simulink library "NMEA"  (R2024a)
settings: Solver=VariableStepAuto  StartTime=0.0  StopTime=10.0  RelTol=1e-3
libraries: $bdroot x44, simulink x21, simulink_extras x17, etargetslib x14
(part 1 of 4)
settings Model: Creator=Scythe  LastModifiedBy=Scythe
settings SolverCC: AlgebraicLoopSolver=TrustRegion
settings DataIOCC: ReturnWorkspaceOutputs=off
settings OptimizationCC: ReuseModelBlockBuffer=off
settings DebuggingCC: UnconnectedInputMsg=warning  UnconnectedOutputMsg=warning  UnconnectedLineMsg=warning  ArithmeticOperatorsInVariantConditions=warning
settings ModelReferenceCC: EnableRefExpFcnMdlSchedulingChecks=on
settings SFSimCC: CustomCodeUndefinedFunction=UseInterfaceOnly
settings RTWCC: GPUComputeCapability=3.5  DLArmComputeVersion=19.05

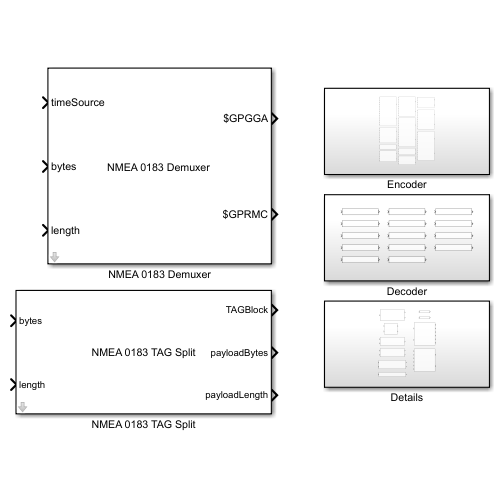
[thumbnail: Simulink's stored preview of the top-level diagram]
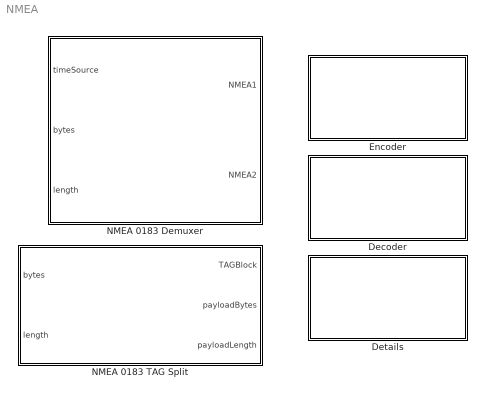
== system NMEA ==
  Decoder : Subsystem
  Details : Subsystem
  Encoder : Subsystem
  NMEA 0183 Demuxer : Subsystem  mask{numMessages=2, idStrings='GPGGA,GPRMC', bufferSize=128, ignoreChecksum=off}
      mask prompts: idStrings "ID strings (separated by comma, e.g: 'GPGGA,GPRMC'):"; bufferSize "Buffer Size (at least 16):"; ignoreChecksum "Ignore Checksum"
      mask help:
      | Receive a binary stream of NMEA 0183 messages and sort them based on the ID. For each ID a separate output port is created. The ID is a string that follows after the start delimiter character.<br><br>
      |
      | <b>timeSource</b><br>
      | The time source to be used to set timestamp values for received messages.<br><br>
      |
      | <b>bytes</b><br>
      | An array of bytes containing binary stream data.<br><br>
      |
      | <b>length</b><br>
      | The length of the actual message in the binary stream data vector.<br><br>
      |
      | <b>OUTPUT PORTS</b><br>
      | An output port is created for each ID string that is specified in the block mask. Each output contains an 8-byte timestamp (double) followed by a buffer containing the actual NMEA message. Thus the output dimension is (8+bufferSize)-by-1. The corresponding output buffer is updated if the checksum is valid or is ignored.
      mask init:
      | % ~~~~~~~~~~~~~~~~~~~~~~~~~~~~~~~~~~~~~~~~~~~~~~~~~~~~~~~~~~~~~~
      | % SETTINGS
      | % ~~~~~~~~~~~~~~~~~~~~~~~~~~~~~~~~~~~~~~~~~~~~~~~~~~~~~~~~~~~~~~
      | portPrefix = 'NMEA';
      | selectorPrefix = 'DataSelector';
      | 
      | 
      | % ~~~~~~~~~~~~~~~~~~~~~~~~~~~~~~~~~~~~~~~~~~~~~~~~~~~~~~~~~~~~~~
      | % Get list of unique IDs and number of messages
      | % ~~~~~~~~~~~~~~~~~~~~~~~~~~~~~~~~~~~~~~~~~~~~~~~~~~~~~~~~~~~~~~
      | listOfIDs = unique(split(char(idStrings),','),'stable');
      | listOfIDs = listOfIDs(~cellfun('isempty',listOfIDs));
      | numMsg = num2str(length(listOfIDs));
      | currentNumMsg = str2num(get_param(gcb,'numMessages'));
      | 
      | 
      | % ~~~~~~~~~~~~~~~~~~~~~~~~~~~~~~~~~~~~~~~~~~~~~~~~~~~~~~~~~~~~~~
      | % Check for unique ID substrings
      | % ~~~~~~~~~~~~~~~~~~~~~~~~~~~~~~~~~~~~~~~~~~~~~~~~~~~~~~~~~~~~~~
      | for i = 1:length(listOfIDs)
      |     for j = 1:length(listOfIDs)
      |         if(i == j), continue; end
      |         if(contains(['$' listOfIDs{i}], ['$' listOfIDs{j}]))
      |             error(['ERROR: ID strings "' listOfIDs{i} '" and "' listOfIDs{j} '" are not unique!']);
      |         end
      |     end
      | end
      | 
      | 
      | % ~~~~~~~~~~~~~~~~~~~~~~~~~~~~~~~~~~~~~~~~~~~~~~~~~~~~~~~~~~~~~~
      | % Only change something if number of messages should be changed
      | % Also check number of current output ports
      | % ~~~~~~~~~~~~~~~~~~~~~~~~~~~~~~~~~~~~~~~~~~~~~~~~~~~~~~~~~~~~~~
      | hThisBlock = get_param(gcb,'PortHandles');
      | if((str2num(numMsg) ~= currentNumMsg) || (length(hThisBlock.Outport) ~= str2num(numMsg)))
      |     % Update parameter
      |     set_param(gcb,'numMessages',numMsg);
      | 
      |     % Handle to demuxer function for signal connection
      |     hDemuxer = get_param([gcb '/Demuxer'],'PortHandles');
      | 
      | 
      |     % ~~~~~~~~~~~~~~~~~~~~~~~~~~~~~~~~~~~~~~~~~~~~~~~~~~~~~~~~~~
      |     % Delete all output ports and selector blocks
      |     % ~~~~~~~~~~~~~~~~~~~~~~~~~~~~~~~~~~~~~~~~~~~~~~~~~~~~~~~~~~
      |     i = 1;
      |     while(true)
      |         % Get names of outport and selector block
      |         outPort = find_system(gcb, 'LookUnderMasks','on','FollowLinks','on','Name',[portPrefix num2str(i)]);
      |         selectorBlock = find_system(gcb, 'LookUnderMasks','on','FollowLinks','on','Name',[selectorPrefix num2str(i)]);
      | 
      |         % Finished if names are empty
      |         if(isempty(outPort) || isempty(selectorBlock))
      |             break;
      |         end
      | 
      |         % Delete lines
      |         outPort = [gcb '/' portPrefix num2str(i)];
      |         selectorBlock = [gcb '/' selectorPrefix num2str(i)];
      |         hOutport = get_param(outPort,'PortHandles');
      |         hSelector = get_param(selectorBlock,'PortHandles');
      |         delete_line(gcb,hSelector.Outport(1),hOutport.Inport(1));
      |         delete_line(gcb,hDemuxer.Outport(1),hSelector.Inport(1));
      | 
      |         % Delete blocks
      |         delete_block(outPort);
      |         delete_block(selectorBlock);
      | 
      |         % Go on with next index
      |         i = i + 1;
      |     end
      | 
      | 
      |     % ~~~~~~~~~~~~~~~~~~~~~~~~~~~~~~~~~~~~~~~~~~~~~~~~~~~~~~~~~~
      |     % Create output ports and selector blocks
      |     % ~~~~~~~~~~~~~~~~~~~~~~~~~~~~~~~~~~~~~~~~~~~~~~~~~~~~~~~~~~
      |     numMsg = get_param(gcb,'numMessages');
      |     N = str2num(numMsg);
      |     for i = 1:N
      |         % Get names of outport and selector block
      |         %outPort = find_system(gcb, 'LookUnderMasks','on','FollowLinks','on','Name',[portPrefix num2str(i)]);
      |         %selectorBlock = find_system(gcb, 'LookUnderMasks','on','FollowLinks','on','Name',[selectorPrefix num2str(i)]);
      |         outPort = [gcb '/' portPrefix num2str(i)];
      |         selectorBlock = [gcb '/' selectorPrefix num2str(i)];
      | 
      |         % Add outport and selector block
      |         add_block('simulink/Ports & Subsystems/Out1',outPort);
      |         add_block('simulink/Signal Routing/Selector',selectorBlock);
      | 
      |         % Set parameters of selector block
      |         set_param(selectorBlock,'IndexMode','One-based','NumberOfDimensions','2','IndexOptions','Select all,Index vector (dialog)','Indices',['[1],' num2str(i)]);
      | 
      |         % Connect selector block to outport
      |         hOutport = get_param(outPort,'PortHandles');
      |         hSelector = get_param(selectorBlock,'PortHandles');
      |         add_line(gcb,hSelector.Outport(1),hOutport.Inport(1));
      | 
      |         % Connect MATLAB function to selector block
      |         add_line(gcb,hDemuxer.Outport(1),hSelector.Inport(1));
      |     end
      | end
      mask DialogControl DescGroupVar Prompt: NMEA 0183 Demuxer
      mask DialogControl group Prompt: Settings
      mask Display:
      | % Get list of unique IDs
      | idStrings = get_param(gcb,'idStrings');
      | idStrings = strrep(idStrings,'''','');
      | listOfIDs = unique(split(char(idStrings),','),'stable');
      | listOfIDs = listOfIDs(~cellfun('isempty',listOfIDs));
      | 
      | % Draw input port labels
      | port_label('input', 1, 'timeSource');
      | port_label('input', 2, 'bytes');
      | port_label('input', 3, 'length');
      | 
      | % Draw output port labels
      | for i = 1:length(listOfIDs)
      |     port_label('output', i, ['$' listOfIDs{i}]);
      | end
      | 
      | % Draw title
      | text(0.5, 0.5, 'NMEA 0183 Demuxer', 'hor', 'center');
  NMEA 0183 TAG Split : Subsystem  mask{ignoreChecksum=off}
      mask prompts: ignoreChecksum "Ignore Checksum"
      mask help:
      | Decodes the <u>first</u> TAG block and outputs all bytes after that TAG block as payload bytes. The input bytes must contain the full message including TAG block and payload. All bytes before the first TAG block are ignored. An NMEA 0183 message with a preceding TAG block (red) looks as follows:<br><br>
      | <span style="color:#f00;">\s:SI0004,n:42*29\</span>[PAYLOAD]<br><br>
      | Here, [PAYLOAD] indicates any NMEA message. The TAG block contains a comma-separated list of code/value pairs.
      | The following parameter codes are supported:
      | <br>
      | <table cellpadding="2" cellspacing="2">
      | 	<tr><th style="background-color: #fff;">Parameter code</th><th style="background-color: #fff;">Description</th></tr>
      | 	<tr><td style="background-color: #ccc;">c</td><td style="background-color: #ccc;">UNIX time</td></tr>
      | 	<tr><td style="background-color: #ddd;">d</td><td style="background-color: #ddd;">Destination ID</td></tr>
      | 	<tr><td style="background-color: #ccc;">g</td><td style="background-color: #ccc;">Grouping</td></tr>
      | 	<tr><td style="background-color: #ddd;">n</td><td style="background-color: #ddd;">Line count</td></tr>
      | 	<tr><td style="background-color: #ccc;">r</td><td style="background-color: #ccc;">Relative time</td></tr>
      | 	<tr><td style="background-color: #ddd;">s</td><td style="background-color: #ddd;">Source ID</td></tr>
      | 	<tr><td style="background-color: #ccc;">t</td><td style="background-color: #ccc;">Text string</td></tr>
      | </table>
      | <br><br>
      | A TAG block ends with an NMEA checksum.
      mask DialogControl DescGroupVar Prompt: NMEA 0183 TAG Split
      mask Display: disp('NMEA 0183 TAG Split')

== system NMEA/Decoder ==
  NMEA 0183 Decode  DPT : Subsystem
      mask help: Decode an NMEA message with ID DPT. The input must be a vector of type uint8 where the first 8 bytes indicate the timestamp and all following bytes indicate the message.
      mask DialogControl DescGroupVar Prompt: NMEA 0183 Decode DPT
  NMEA 0183 Decode ALR : Subsystem
      mask help: Decode an NMEA message with ID ALR. The input must be a vector of type uint8 where the first 8 bytes indicate the timestamp and all following bytes indicate the message.
      mask DialogControl DescGroupVar Prompt: NMEA 0183 Decode ALR
  NMEA 0183 Decode DBT : Subsystem
      mask help: Decode an NMEA message with ID DBT. The input must be a vector of type uint8 where the first 8 bytes indicate the timestamp and all following bytes indicate the message.
      mask DialogControl DescGroupVar Prompt: NMEA 0183 Decode DBT
  NMEA 0183 Decode GGA : Subsystem
      mask help: Decode an NMEA message with ID GGA. The input must be a vector of type uint8 where the first 8 bytes indicate the timestamp and all following bytes indicate the message.
      mask DialogControl DescGroupVar Prompt: NMEA 0183 Decode GGA
  NMEA 0183 Decode HDT : Subsystem
      mask help: Decode an NMEA message with ID HDT. The input must be a vector of type uint8 where the first 8 bytes indicate the timestamp and all following bytes indicate the message.
      mask DialogControl DescGroupVar Prompt: NMEA 0183 Decode HDT
  NMEA 0183 Decode MDA : Subsystem
      mask help: Decode an NMEA message with ID MDA. The input must be a vector of type uint8 where the first 8 bytes indicate the timestamp and all following bytes indicate the message.
      mask DialogControl DescGroupVar Prompt: NMEA 0183 Decode MDA
  NMEA 0183 Decode MWV : Subsystem
      mask help: Decode an NMEA message with ID MWV. The input must be a vector of type uint8 where the first 8 bytes indicate the timestamp and all following bytes indicate the message.
      mask DialogControl DescGroupVar Prompt: NMEA 0183 Decode MWV
  NMEA 0183 Decode RMC : Subsystem
      mask help: Decode an NMEA message with ID RMC. The input must be a vector of type uint8 where the first 8 bytes indicate the timestamp and all following bytes indicate the message.
      mask DialogControl DescGroupVar Prompt: NMEA 0183 Decode RMC
  NMEA 0183 Decode RMC Extended : Subsystem
      mask help: Decode an NMEA message with ID RMC (extended version). The input must be a vector of type uint8 where the first 8 bytes indicate the timestamp and all following bytes indicate the message.
      mask DialogControl DescGroupVar Prompt: NMEA 0183 Decode RMC Extended
  NMEA 0183 Decode ROT : Subsystem
      mask help: Decode an NMEA message with ID ROT. The input must be a vector of type uint8 where the first 8 bytes indicate the timestamp and all following bytes indicate the message.
      mask DialogControl DescGroupVar Prompt: NMEA 0183 Decode ROT
  NMEA 0183 Decode VBW : Subsystem
      mask help: Decode an NMEA message with ID VBW. The input must be a vector of type uint8 where the first 8 bytes indicate the timestamp and all following bytes indicate the message.
      mask DialogControl DescGroupVar Prompt: NMEA 0183 Decode VBW
  NMEA 0183 Decode VTG : Subsystem
      mask help: Decode an NMEA message with ID VTG. The input must be a vector of type uint8 where the first 8 bytes indicate the timestamp and all following bytes indicate the message.
      mask DialogControl DescGroupVar Prompt: NMEA 0183 Decode VTG
  NMEA 0183 Decode XDR16 : Subsystem
      mask help: Decode XDR messages. XDR messages have a variable number of fields. This decoder can decode 16 fields. Each field has a type (1 byte), unit (1 byte), value (1 double) and name (4 bytes).
      mask DialogControl DescGroupVar Prompt: NMEA 0183 Decode XDR16
      mask Display: disp('NMEA 0183 Decode XDR\n(16)')
  NMEA 0183 Decode ZDA : Subsystem
      mask help: Decode an NMEA message with ID ZDA. The input must be a vector of type uint8 where the first 8 bytes indicate the timestamp and all following bytes indicate the message.
      mask DialogControl DescGroupVar Prompt: NMEA 0183 Decode ZDA

== system NMEA/Details ==
  Append CR LF : Subsystem
      mask help: Append two bytes (&lt;CR&gt;&lt;LF&gt;) at the end of the input buffer. Both bytes are only assigned to the input buffer if the input length indicates a free memory of at least two bytes.
      mask DialogControl DescGroupVar Prompt: Append CR LF
  Ensure Positive Angle : Subsystem
      mask help: Convert a given angle [rad] to an output angle [rad] with the output angle being in range [0, +2*pi).
      mask DialogControl DescGroupVar Prompt: Ensure Symmetrical Angle
      mask Display:
      | % Get dimension of block
      | pos = get_param(gcb, 'Position');
      | width = pos(3) - pos(1);
      | height = pos(4) - pos(2);
      | 
      | % Set equation
      | text(0.5*width,0.5*height,'[0, +2\pi)', 'hor','center','texmode','on');
  Ensure Symmetrical Angle : Subsystem
      mask help: Convert a given angle [rad] to an output angle [rad] with the output angle being in range [-pi, +pi).
      mask DialogControl DescGroupVar Prompt: Ensure Symmetrical Angle
      mask Display:
      | % Get dimension of block
      | pos = get_param(gcb, 'Position');
      | width = pos(3) - pos(1);
      | height = pos(4) - pos(2);
      | 
      | % Set equation
      | text(0.5*width,0.5*height,'[-\pi, +\pi)', 'hor','center','texmode','on');
  NMEA Checksum Message : Subsystem
      mask help:
      | Create an NMEA message including the checksum.<br><br>
      | <b>INPUT</b><br>
      | <b>nmeaString</b><br>
      | The NMEA string including the dollar-delimiter at the beginning and the '*'-character at the end.<br><br>
      |
      | <b>OUTPUT</b><br>
      | <b>bytes</b><br>
      | Bytes of the NMEA message containing the input string and the checksum. CR-LF is not added. The output buffer size is 128 bytes.<br><br>
      |
      | <b>length</b><br>
      | The actual length of the message in the output buffer.<br><br>
      mask DialogControl DescGroupVar Prompt: NMEA Checksum Message
      mask Display: disp('NMEA\nChecksum Message');
  NMEA Checksum Test : Subsystem
      mask help: Check whether the checksum of the <u>first</u> NMEA message is correct or not.
      mask DialogControl DescGroupVar Prompt: NMEA Checksum Test
      mask Display: disp('NMEA Checksum Test');
  NMEA Decode Position : Subsystem
      mask help: Decode (parse) geographic position from NMEA representation.
      mask DialogControl DescGroupVar Prompt: NMEA Decode Position
      mask Display: disp('NMEA Decode Position');
  NMEA Encode Position : Subsystem
      mask help: Encode a geographic position to a corresponding NMEA representation.
      mask DialogControl DescGroupVar Prompt: NMEA Encode Position
      mask Display: disp('NMEA Encode Position');
  NMEA Fill Empty Fields : Subsystem
      mask help:
      | Fill empty fields with zeros. ",," is replaced by ",0," and ",*" is replaced by ",0*". This is helpful for subsequent string scan operations to work. <br><br>
      | <b>Note:</b> The checksum is not updated!
      mask DialogControl DescGroupVar Prompt: NMEA Fill Empty Fields
      mask Display: disp('NMEA Fill Empty Fields');
  NMEA XDR16 Get Value Of Transducer : Subsystem
      mask help: Get the value for a given transducer name (4 bytes). If this name was not found, the value output is zero and the found output is false.
      mask DialogControl DescGroupVar Prompt: NMEA XDR16 Get Value Of Transducer
      mask Display: disp('NMEA XDR16 Get Value Of Transducer')
  Select NMEA and Fill Empty Fields : Subsystem
      mask help: Select the NMEA message from the input <b>Timestamp_NMEA</b> (the first 8 bytes indicate the timestamp) and fill empty fields by zeros. For example, "A,B,,,,C" becomes "A,B,0,0,0,C".
      mask DialogControl DescGroupVar Prompt: Select NMEA and Fill Empty Fields
      mask Display: disp('Select NMEA\nFill Empty Fields')

== system NMEA/Encoder ==
  NMEA 0183 Encode ALR : Subsystem
      mask help: Encode an NMEA message with ID ALR. The output buffer size is 128 bytes. The length output indicates the actual length of the message.
      mask DialogControl DescGroupVar Prompt: NMEA 0183 Encode ALR
  NMEA 0183 Encode DBT : Subsystem
      mask help: Encode an NMEA message with ID DBT. The output buffer size is 128 bytes. The length output indicates the actual length of the message.
      mask DialogControl DescGroupVar Prompt: NMEA 0183 Encode DBT
  NMEA 0183 Encode GGA : Subsystem
      mask help: Encode an NMEA message with ID GGA. The output buffer size is 128 bytes. The length output indicates the actual length of the message.
      mask DialogControl DescGroupVar Prompt: NMEA 0183 Encode GGA
  NMEA 0183 Encode HDT : Subsystem
      mask help: Encode an NMEA message with ID HDT. The output buffer size is 128 bytes. The length output indicates the actual length of the message.
      mask DialogControl DescGroupVar Prompt: NMEA 0183 Encode HDT
  NMEA 0183 Encode MWV : Subsystem
      mask help: Encode an NMEA message with ID MWV. The output buffer size is 128 bytes. The length output indicates the actual length of the message.
      mask DialogControl DescGroupVar Prompt: NMEA 0183 Encode MWV
  NMEA 0183 Encode RMC : Subsystem
      mask help: Encode an NMEA message with ID RMC. The output buffer size is 128 bytes. The length output indicates the actual length of the message.
      mask DialogControl DescGroupVar Prompt: NMEA 0183 Encode RMC
  NMEA 0183 Encode RMC Extended : Subsystem
      mask help: Encode an NMEA message with ID RMC (extended message type). The output buffer size is 128 bytes. The length output indicates the actual length of the message.
      mask DialogControl DescGroupVar Prompt: NMEA 0183 Encode RMC Extended
  NMEA 0183 Encode ROT : Subsystem
      mask help: Encode an NMEA message with ID ROT. The output buffer size is 128 bytes. The length output indicates the actual length of the message.
      mask DialogControl DescGroupVar Prompt: NMEA 0183 Encode ROT
  NMEA 0183 Encode VBW : Subsystem
      mask help: Encode an NMEA message with ID VBW. The output buffer size is 128 bytes. The length output indicates the actual length of the message.
      mask DialogControl DescGroupVar Prompt: NMEA 0183 Encode VBW
  NMEA 0183 Encode VTG : Subsystem
      mask help: Encode an NMEA message with ID VTG. The output buffer size is 128 bytes. The length output indicates the actual length of the message.
      mask DialogControl DescGroupVar Prompt: NMEA 0183 Encode VTG
  NMEA 0183 Encode ZDA : Subsystem
      mask help: Encode an NMEA message with ID ZDA. The output buffer size is 128 bytes. The length output indicates the actual length of the message.
      mask DialogControl DescGroupVar Prompt: NMEA 0183 Encode ZDA

== system NMEA/NMEA 0183 Demuxer ==
  timeSource : Inport  OutDataTypeStr=double  Unit=s  PortDimensions=1
  bytes : Inport  Port=2  OutDataTypeStr=uint8
  length : Inport  Port=3  OutDataTypeStr=uint32  PortDimensions=1
  Constant : Constant  Value=uint8(idStrings)
  Data Type Conversion : DataTypeConversion  OutDataTypeStr=int32  SaturateOnIntegerOverflow=off  RndMeth=Floor
  DataSelector1 : Selector  NumberOfDimensions=2  InputPortWidth=3  IndexOptions=Select all,Index vector (dialog)  Indices=[1],1  OutputSizes=1
  DataSelector2 : Selector  NumberOfDimensions=2  InputPortWidth=3  IndexOptions=Select all,Index vector (dialog)  Indices=[1],2  OutputSizes=1
  Demuxer : MATLAB Function  TreatAsAtomicUnit=on
  NMEA1 : Outport
  NMEA2 : Outport  Port=2
  wires:
  timeSource/1 -> Demuxer/1(timeSource)
  bytes/1 -> Demuxer/2(bytes)
  length/1 -> Data Type Conversion/1
  Data Type Conversion/1 -> Demuxer/3(len)
  Constant/1 -> Demuxer/4(idStrings)
  DataSelector1/1 -> NMEA1/1
  Demuxer/1(messages) -> DataSelector1/1, DataSelector2/1
  DataSelector2/1 -> NMEA2/1

== system NMEA/NMEA 0183 TAG Split ==
  bytes : Inport  OutDataTypeStr=uint8
  length : Inport  Port=2  OutDataTypeStr=uint32  PortDimensions=1
  Bus Creator : BusCreator  Inputs=7
  MATLAB Function : MATLAB Function  TreatAsAtomicUnit=on
  TAGBlock : Outport
  payloadBytes : Outport  Port=2  OutDataTypeStr=uint8
  payloadLength : Outport  Port=3  OutDataTypeStr=uint32  PortDimensions=1
  wires:
  bytes/1 -> MATLAB Function/1(bytes)
  MATLAB Function/1(tag_c) -> Bus Creator/1  "c"
  MATLAB Function/5(tag_r) -> Bus Creator/5  "r"
  MATLAB Function/4(tag_n) -> Bus Creator/4  "n"
  MATLAB Function/7(tag_t) -> Bus Creator/7  "t"
  MATLAB Function/3(tag_g) -> Bus Creator/3  "g"
  MATLAB Function/2(tag_d) -> Bus Creator/2  "d"
  MATLAB Function/6(tag_s) -> Bus Creator/6  "s"
  Bus Creator/1 -> TAGBlock/1
  length/1 -> MATLAB Function/2(len)
  MATLAB Function/8(payloadBytes) -> payloadBytes/1
  MATLAB Function/9(payloadLength) -> payloadLength/1

== system NMEA/Decoder/NMEA 0183 Decode  DPT ==
  Timestamp_NMEA : Inport
  ASCII to String3 : ASCIIToString
  Byte Unpack2 : etargetslib/Byte Unpack  dimensions={1}  datatypes={'double'}  byteAlign=1
  Compare To Constant : simulink/Logic and Bit Operations/Compare To Constant  relop===  const=uint8(42)  OutDataTypeStr=boolean
  DecodeMessage : Subsystem  TreatAsAtomicUnit=on
  Scan String : ScanString  Format="\"$%c%cDPT,%lf,%lf,%lf%c\""
  Select NMEA and Fill Empty Fields : $bdroot/Details/Select NMEA and Fill Empty Fields
  SelectTimestamp : Selector  IndexOptions=Index vector (dialog)  Indices=1:8  OutputSizes=1
  String Concatenate : StringConcatenate
  String to ASCII : StringToASCII  OutputVectorSize=1
  DPT : Outport
  wires:
  Compare To Constant/1 -> DecodeMessage/Enable
  Scan String/2 -> String Concatenate/2
  String Concatenate/1 -> DecodeMessage/2(strID)
  ASCII to String3/1 -> Scan String/1
  Timestamp_NMEA/1 -> SelectTimestamp/1, Select NMEA and Fill Empty Fields/1
  DecodeMessage/1(DPT) -> DPT/1
  Byte Unpack2/1 -> DecodeMessage/1(timestamp)  "timestamp"
  SelectTimestamp/1 -> Byte Unpack2/1
  String to ASCII/1 -> Compare To Constant/1
  Select NMEA and Fill Empty Fields/1 -> ASCII to String3/1
  Scan String/1 -> String Concatenate/1
  Scan String/6 -> String to ASCII/1
  Scan String/3 -> DecodeMessage/3(depth)
  Scan String/4 -> DecodeMessage/4(offset)
  Scan String/5 -> DecodeMessage/5(range)

== system NMEA/Decoder/NMEA 0183 Decode ALR ==
  Timestamp_NMEA : Inport
  ASCII to String3 : ASCIIToString
  Byte Unpack2 : etargetslib/Byte Unpack  dimensions={1}  datatypes={'double'}  byteAlign=1
  DecodeMessage : Subsystem  TreatAsAtomicUnit=on
  Scan String : ScanString  Format="\"$%c%cALR,%02u%02u%lf,%1u%1u%1u,%c,%c,%s\""
  Select NMEA and Fill Empty Fields : $bdroot/Details/Select NMEA and Fill Empty Fields
  SelectTimestamp : Selector  IndexOptions=Index vector (dialog)  Indices=1:8  OutputSizes=1
  String Concatenate : StringConcatenate
  String Constant : StringConstant  String="\"*\""
  String Contains : StringContains
  ALR : Outport
  wires:
  Scan String/2 -> String Concatenate/2
  String Concatenate/1 -> DecodeMessage/2(strID)
  ASCII to String3/1 -> Scan String/1
  Timestamp_NMEA/1 -> Select NMEA and Fill Empty Fields/1, SelectTimestamp/1
  DecodeMessage/1(ALR) -> ALR/1
  Byte Unpack2/1 -> DecodeMessage/1(timestamp)  "timestamp"
  SelectTimestamp/1 -> Byte Unpack2/1
  Select NMEA and Fill Empty Fields/1 -> ASCII to String3/1
  Scan String/1 -> String Concatenate/1
  String Constant/1 -> String Contains/2
  Scan String/11 -> String Contains/1
  String Contains/1 -> DecodeMessage/Enable
  Scan String/3 -> DecodeMessage/3(utcHour)
  Scan String/5 -> DecodeMessage/5(utcSecond)
  Scan String/4 -> DecodeMessage/4(utcMinute)
  Scan String/7 -> DecodeMessage/7(alarmID2)
  Scan String/8 -> DecodeMessage/8(alarmID3)
  Scan String/9 -> DecodeMessage/9(strAlarmCondition)
  Scan String/10 -> DecodeMessage/10(strAlarmAcknowledge)
  Scan String/6 -> DecodeMessage/6(alarmID1)

== system NMEA/Decoder/NMEA 0183 Decode DBT ==
  Timestamp_NMEA : Inport
  ASCII to String3 : ASCIIToString
  Byte Unpack2 : etargetslib/Byte Unpack  dimensions={1}  datatypes={'double'}  byteAlign=1
  Compare To Constant : simulink/Logic and Bit Operations/Compare To Constant  relop===  const=uint8(42)  OutDataTypeStr=boolean
  DecodeMessage : Subsystem  TreatAsAtomicUnit=on
  Scan String : ScanString  Format="\"$%c%cDBT,%lf,f,%lf,M,%lf,F%c\""
  Select NMEA and Fill Empty Fields : $bdroot/Details/Select NMEA and Fill Empty Fields
  SelectTimestamp : Selector  IndexOptions=Index vector (dialog)  Indices=1:8  OutputSizes=1
  String Concatenate : StringConcatenate
  String to ASCII : StringToASCII  OutputVectorSize=1
  DBT : Outport
  wires:
  Scan String/6 -> String to ASCII/1
  Scan String/5 -> DecodeMessage/5(depthFathoms)
  Scan String/4 -> DecodeMessage/4(depthMeters)
  Scan String/3 -> DecodeMessage/3(depthFeet)
  Compare To Constant/1 -> DecodeMessage/Enable
  Scan String/2 -> String Concatenate/2
  String Concatenate/1 -> DecodeMessage/2(strID)
  ASCII to String3/1 -> Scan String/1
  Timestamp_NMEA/1 -> Select NMEA and Fill Empty Fields/1, SelectTimestamp/1
  DecodeMessage/1(DBT) -> DBT/1
  Byte Unpack2/1 -> DecodeMessage/1(timestamp)  "timestamp"
  SelectTimestamp/1 -> Byte Unpack2/1
  String to ASCII/1 -> Compare To Constant/1
  Select NMEA and Fill Empty Fields/1 -> ASCII to String3/1
  Scan String/1 -> String Concatenate/1

== system NMEA/Decoder/NMEA 0183 Decode GGA ==
  Timestamp_NMEA : Inport
  ASCII to String3 : ASCIIToString
  Byte Unpack2 : etargetslib/Byte Unpack  dimensions={1}  datatypes={'double'}  byteAlign=1
  Compare To Constant : simulink/Logic and Bit Operations/Compare To Constant  relop===  const=uint8(42)  OutDataTypeStr=boolean
  DecodeMessage : Subsystem  TreatAsAtomicUnit=on
  Scan String : ScanString  Format="\"$%c%cGGA,%02u%02u%lf,%02u%lf,%c,%03u%lf,%c,%u,%u,%lf,%lf,M,%lf,M,%lf,%u%c\""
  Select NMEA and Fill Empty Fields : $bdroot/Details/Select NMEA and Fill Empty Fields
  SelectTimestamp : Selector  IndexOptions=Index vector (dialog)  Indices=1:8  OutputSizes=1
  String Concatenate : StringConcatenate
  String to ASCII : StringToASCII  OutputVectorSize=1
  GGA : Outport
  wires:
  Scan String/8 -> DecodeMessage/8(strLatSign)
  Scan String/1 -> String Concatenate/1
  Select NMEA and Fill Empty Fields/1 -> ASCII to String3/1
  Scan String/5 -> DecodeMessage/5(utcSecond)
  String to ASCII/1 -> Compare To Constant/1
  Scan String/3 -> DecodeMessage/3(utcHour)
  SelectTimestamp/1 -> Byte Unpack2/1
  Scan String/19 -> String to ASCII/1
  Scan String/9 -> DecodeMessage/9(lonDeg)
  Byte Unpack2/1 -> DecodeMessage/1(timestamp)  "timestamp"
  Scan String/12 -> DecodeMessage/12(gpsQuality)
  DecodeMessage/1(GGA) -> GGA/1
  Timestamp_NMEA/1 -> Select NMEA and Fill Empty Fields/1, SelectTimestamp/1
  Scan String/11 -> DecodeMessage/11(strLonSign)
  Scan String/15 -> DecodeMessage/15(antennaHeightMSL)
  Scan String/6 -> DecodeMessage/6(latDeg)
  ASCII to String3/1 -> Scan String/1
  String Concatenate/1 -> DecodeMessage/2(strID)
  Scan String/4 -> DecodeMessage/4(utcMinute)
  Scan String/7 -> DecodeMessage/7(latMin)
  Scan String/2 -> String Concatenate/2
  Scan String/13 -> DecodeMessage/13(numSat)
  Scan String/10 -> DecodeMessage/10(lonMin)
  Compare To Constant/1 -> DecodeMessage/Enable
  Scan String/14 -> DecodeMessage/14(hdop)
  Scan String/16 -> DecodeMessage/16(geoidSeparation)
  Scan String/17 -> DecodeMessage/17(ageOfDGPS)
  Scan String/18 -> DecodeMessage/18(dgpsReferenceStation)

== system NMEA/Decoder/NMEA 0183 Decode HDT ==
  Timestamp_NMEA : Inport
  ASCII to String3 : ASCIIToString
  Byte Unpack2 : etargetslib/Byte Unpack  dimensions={1}  datatypes={'double'}  byteAlign=1
  Compare To Constant : simulink/Logic and Bit Operations/Compare To Constant  relop===  const=uint8(42)  OutDataTypeStr=boolean
  DecodeMessage : Subsystem  TreatAsAtomicUnit=on
  Scan String : ScanString  Format="\"$%c%cHDT,%lf,T%c\""
  Select NMEA and Fill Empty Fields : $bdroot/Details/Select NMEA and Fill Empty Fields
  SelectTimestamp : Selector  IndexOptions=Index vector (dialog)  Indices=1:8  OutputSizes=1
  String Concatenate : StringConcatenate
  String to ASCII : StringToASCII  OutputVectorSize=1
  HDT : Outport
  wires:
  Scan String/4 -> String to ASCII/1
  Scan String/1 -> String Concatenate/1
  Select NMEA and Fill Empty Fields/1 -> ASCII to String3/1
  String to ASCII/1 -> Compare To Constant/1
  SelectTimestamp/1 -> Byte Unpack2/1
  Byte Unpack2/1 -> DecodeMessage/1(timestamp)  "timestamp"
  DecodeMessage/1(HDT) -> HDT/1
  Timestamp_NMEA/1 -> Select NMEA and Fill Empty Fields/1, SelectTimestamp/1
  ASCII to String3/1 -> Scan String/1
  String Concatenate/1 -> DecodeMessage/2(strID)
  Scan String/2 -> String Concatenate/2
  Compare To Constant/1 -> DecodeMessage/Enable
  Scan String/3 -> DecodeMessage/3(trueHeading)

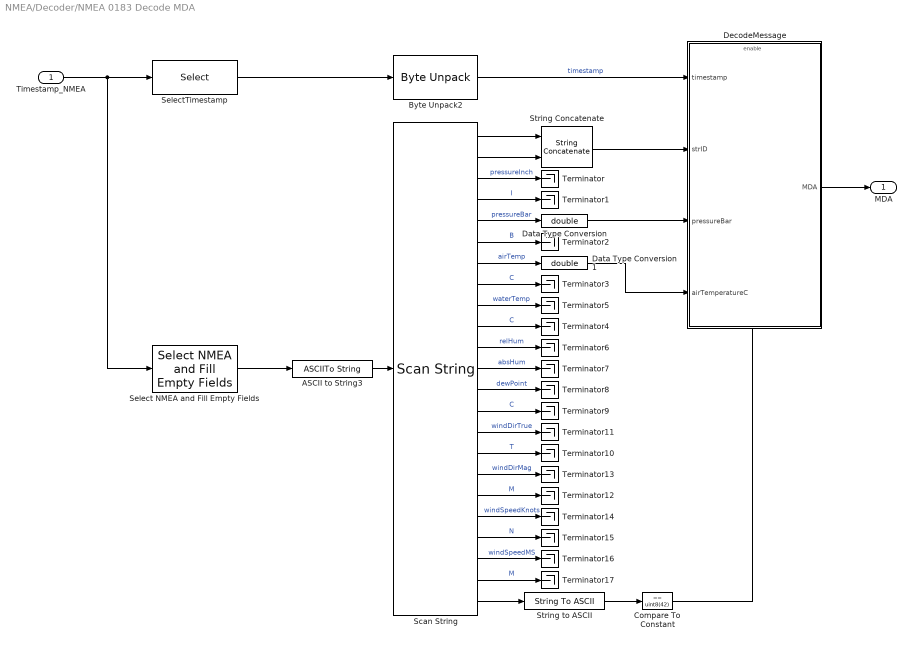
== system NMEA/Decoder/NMEA 0183 Decode MDA ==
  Timestamp_NMEA : Inport
  ASCII to String3 : ASCIIToString
  Byte Unpack2 : etargetslib/Byte Unpack  dimensions={1}  datatypes={'double'}  byteAlign=1
  Compare To Constant : simulink/Logic and Bit Operations/Compare To Constant  relop===  const=uint8(42)  OutDataTypeStr=boolean
  Data Type Conversion : DataTypeConversion  OutDataTypeStr=double  SaturateOnIntegerOverflow=off  RndMeth=Floor
  Data Type Conversion1 : DataTypeConversion  OutDataTypeStr=double  SaturateOnIntegerOverflow=off  RndMeth=Floor
  DecodeMessage : Subsystem  TreatAsAtomicUnit=on
  Scan String : ScanString  Format="\"$%c%cMDA,%lf,%c,%lf,%c,%lf,%c,%lf,%c,%lf,%lf,%lf,%c,%lf,%c,%lf,%c,%lf,%c,%lf,%c%c\""
  Select NMEA and Fill Empty Fields : $bdroot/Details/Select NMEA and Fill Empty Fields
  SelectTimestamp : Selector  IndexOptions=Index vector (dialog)  Indices=1:8  OutputSizes=1
  String Concatenate : StringConcatenate
  String to ASCII : StringToASCII  OutputVectorSize=1
  Terminator{,1..17} (18 alike) : Terminator
  MDA : Outport
  wires:
  Compare To Constant/1 -> DecodeMessage/Enable
  Scan String/2 -> String Concatenate/2
  String Concatenate/1 -> DecodeMessage/2(strID)
  ASCII to String3/1 -> Scan String/1
  Timestamp_NMEA/1 -> Select NMEA and Fill Empty Fields/1, SelectTimestamp/1
  DecodeMessage/1(MDA) -> MDA/1
  Byte Unpack2/1 -> DecodeMessage/1(timestamp)  "timestamp"
  SelectTimestamp/1 -> Byte Unpack2/1
  String to ASCII/1 -> Compare To Constant/1
  Select NMEA and Fill Empty Fields/1 -> ASCII to String3/1
  Scan String/1 -> String Concatenate/1
  Scan String/23 -> String to ASCII/1
  Scan String/3 -> Terminator/1  "pressureInch"
  Scan String/4 -> Terminator1/1  "I"
  Scan String/5 -> Data Type Conversion/1  "pressureBar"
  Scan String/6 -> Terminator2/1  "B"
  Scan String/7 -> Data Type Conversion1/1  "airTemp"
  Scan String/8 -> Terminator3/1  "C"
  Scan String/9 -> Terminator5/1  "waterTemp"
  Scan String/10 -> Terminator4/1  "C"
  Scan String/11 -> Terminator6/1  "relHum"
  Scan String/12 -> Terminator7/1  "absHum"
  Scan String/13 -> Terminator8/1  "dewPoint"
  Scan String/14 -> Terminator9/1  "C"
  Scan String/15 -> Terminator11/1  "windDirTrue"
  Scan String/16 -> Terminator10/1  "T"
  Scan String/18 -> Terminator12/1  "M"
  Scan String/17 -> Terminator13/1  "windDirMag"
  Scan String/19 -> Terminator14/1  "windSpeedKnots"
  Scan String/20 -> Terminator15/1  "N"
  Scan String/21 -> Terminator16/1  "windSpeedMS"
  Scan String/22 -> Terminator17/1  "M"
  Data Type Conversion/1 -> DecodeMessage/3(pressureBar)
  Data Type Conversion1/1 -> DecodeMessage/4(airTemperatureC)

== system NMEA/Decoder/NMEA 0183 Decode MWV ==
  Timestamp_NMEA : Inport
  ASCII to String3 : ASCIIToString
  Byte Unpack2 : etargetslib/Byte Unpack  dimensions={1}  datatypes={'double'}  byteAlign=1
  Compare To Constant : simulink/Logic and Bit Operations/Compare To Constant  relop===  const=uint8(42)  OutDataTypeStr=boolean
  DecodeMessage : Subsystem  TreatAsAtomicUnit=on
  Scan String : ScanString  Format="\"$%c%cMWV,%lf,%c,%lf,%c,%c%c\""
  Select NMEA and Fill Empty Fields : $bdroot/Details/Select NMEA and Fill Empty Fields
  SelectTimestamp : Selector  IndexOptions=Index vector (dialog)  Indices=1:8  OutputSizes=1
  String Concatenate : StringConcatenate
  String to ASCII : StringToASCII  OutputVectorSize=1
  MWV : Outport
  wires:
  Scan String/1 -> String Concatenate/1
  Select NMEA and Fill Empty Fields/1 -> ASCII to String3/1
  String to ASCII/1 -> Compare To Constant/1
  SelectTimestamp/1 -> Byte Unpack2/1
  Byte Unpack2/1 -> DecodeMessage/1(timestamp)  "timestamp"
  DecodeMessage/1(MWV) -> MWV/1
  Timestamp_NMEA/1 -> Select NMEA and Fill Empty Fields/1, SelectTimestamp/1
  ASCII to String3/1 -> Scan String/1
  String Concatenate/1 -> DecodeMessage/2(strID)
  Scan String/2 -> String Concatenate/2
  Compare To Constant/1 -> DecodeMessage/Enable
  Scan String/3 -> DecodeMessage/3(windAngle)
  Scan String/8 -> String to ASCII/1
  Scan String/4 -> DecodeMessage/4(strWindAngleReference)
  Scan String/5 -> DecodeMessage/5(windSpeed)
  Scan String/6 -> DecodeMessage/6(strWindSpeedUnit)
  Scan String/7 -> DecodeMessage/7(strStatus)

== system NMEA/Decoder/NMEA 0183 Decode RMC ==
  Timestamp_NMEA : Inport
  ASCII to String3 : ASCIIToString
  Byte Unpack2 : etargetslib/Byte Unpack  dimensions={1}  datatypes={'double'}  byteAlign=1
  Compare To Constant : simulink/Logic and Bit Operations/Compare To Constant  relop===  const=uint8(42)  OutDataTypeStr=boolean
  DecodeMessage : Subsystem  TreatAsAtomicUnit=on
  Scan String : ScanString  Format="\"$%c%cRMC,%02u%02u%lf,%c,%02u%lf,%c,%03u%lf,%c,%lf,%lf,%02u%02u%02u,%lf,%c%c\""
  Select NMEA and Fill Empty Fields : $bdroot/Details/Select NMEA and Fill Empty Fields
  SelectTimestamp : Selector  IndexOptions=Index vector (dialog)  Indices=1:8  OutputSizes=1
  String Concatenate : StringConcatenate
  String to ASCII : StringToASCII  OutputVectorSize=1
  RMC : Outport
  wires:
  Compare To Constant/1 -> DecodeMessage/Enable
  Scan String/2 -> String Concatenate/2
  Scan String/4 -> DecodeMessage/4(utcMinute)
  String Concatenate/1 -> DecodeMessage/2(strID)
  ASCII to String3/1 -> Scan String/1
  Timestamp_NMEA/1 -> Select NMEA and Fill Empty Fields/1, SelectTimestamp/1
  DecodeMessage/1(RMC) -> RMC/1
  Byte Unpack2/1 -> DecodeMessage/1(timestamp)  "timestamp"
  Scan String/20 -> String to ASCII/1
  SelectTimestamp/1 -> Byte Unpack2/1
  Scan String/3 -> DecodeMessage/3(utcHour)
  String to ASCII/1 -> Compare To Constant/1
  Select NMEA and Fill Empty Fields/1 -> ASCII to String3/1
  Scan String/1 -> String Concatenate/1
  Scan String/5 -> DecodeMessage/5(utcSecond)
  Scan String/6 -> DecodeMessage/6(strStatus)
  Scan String/7 -> DecodeMessage/7(latDeg)
  Scan String/8 -> DecodeMessage/8(latMin)
  Scan String/9 -> DecodeMessage/9(strLatSign)
  Scan String/10 -> DecodeMessage/10(lonDeg)
  Scan String/11 -> DecodeMessage/11(lonMin)
  Scan String/12 -> DecodeMessage/12(strLonSign)
  Scan String/13 -> DecodeMessage/13(speedOverGround)
  Scan String/14 -> DecodeMessage/14(courseOverGround)
  Scan String/15 -> DecodeMessage/15(dateDay)
  Scan String/16 -> DecodeMessage/16(dateMonth)
  Scan String/17 -> DecodeMessage/17(dateYear)
  Scan String/18 -> DecodeMessage/18(magneticVariation)
  Scan String/19 -> DecodeMessage/19(strMagneticVariationSign)

== system NMEA/Decoder/NMEA 0183 Decode RMC Extended ==
  Timestamp_NMEA : Inport
  ASCII to String3 : ASCIIToString
  Byte Unpack2 : etargetslib/Byte Unpack  dimensions={1}  datatypes={'double'}  byteAlign=1
  Compare To Constant : simulink/Logic and Bit Operations/Compare To Constant  relop===  const=uint8(42)  OutDataTypeStr=boolean
  DecodeMessage : Subsystem  TreatAsAtomicUnit=on
  Scan String : ScanString  Format="\"$%c%cRMC,%02u%02u%lf,%c,%02u%lf,%c,%03u%lf,%c,%lf,%lf,%02u%02u%02u,%lf,%lf,%c,V%c\""
  Select NMEA and Fill Empty Fields : $bdroot/Details/Select NMEA and Fill Empty Fields
  SelectTimestamp : Selector  IndexOptions=Index vector (dialog)  Indices=1:8  OutputSizes=1
  String Concatenate : StringConcatenate
  String to ASCII : StringToASCII  OutputVectorSize=1
  Terminator2 : Terminator
  Terminator3 : Terminator
  RMC : Outport
  wires:
  Byte Unpack2/1 -> DecodeMessage/1(timestamp)  "timestamp"
  Scan String/21 -> String to ASCII/1
  Scan String/19 -> Terminator2/1
  Scan String/17 -> DecodeMessage/17(dateYear)
  Scan String/16 -> DecodeMessage/16(dateMonth)
  Scan String/15 -> DecodeMessage/15(dateDay)
  Scan String/14 -> DecodeMessage/14(courseOverGround)
  Scan String/13 -> DecodeMessage/13(speedOverGround)
  Scan String/12 -> DecodeMessage/12(strLonSign)
  Scan String/11 -> DecodeMessage/11(lonMin)
  Scan String/10 -> DecodeMessage/10(lonDeg)
  Scan String/9 -> DecodeMessage/9(strLatSign)
  Scan String/8 -> DecodeMessage/8(latMin)
  Scan String/7 -> DecodeMessage/7(latDeg)
  Scan String/6 -> DecodeMessage/6(strStatus)
  Scan String/5 -> DecodeMessage/5(utcSecond)
  Scan String/1 -> String Concatenate/1
  String to ASCII/1 -> Compare To Constant/1
  Scan String/3 -> DecodeMessage/3(utcHour)
  String Concatenate/1 -> DecodeMessage/2(strID)
  Scan String/4 -> DecodeMessage/4(utcMinute)
  Scan String/2 -> String Concatenate/2
  Compare To Constant/1 -> DecodeMessage/Enable
  Scan String/18 -> Terminator3/1
  Scan String/20 -> DecodeMessage/18(strMode)
  Select NMEA and Fill Empty Fields/1 -> ASCII to String3/1
  SelectTimestamp/1 -> Byte Unpack2/1
  DecodeMessage/1(RMC) -> RMC/1
  Timestamp_NMEA/1 -> Select NMEA and Fill Empty Fields/1, SelectTimestamp/1
  ASCII to String3/1 -> Scan String/1

== system NMEA/Decoder/NMEA 0183 Decode ROT ==
  Timestamp_NMEA : Inport
  ASCII to String3 : ASCIIToString
  Byte Unpack2 : etargetslib/Byte Unpack  dimensions={1}  datatypes={'double'}  byteAlign=1
  Compare To Constant : simulink/Logic and Bit Operations/Compare To Constant  relop===  const=uint8(42)  OutDataTypeStr=boolean
  DecodeMessage : Subsystem  TreatAsAtomicUnit=on
  Scan String : ScanString  Format="\"$%c%cROT,%lf,%c%c\""
  Select NMEA and Fill Empty Fields : $bdroot/Details/Select NMEA and Fill Empty Fields
  SelectTimestamp : Selector  IndexOptions=Index vector (dialog)  Indices=1:8  OutputSizes=1
  String Concatenate : StringConcatenate
  String to ASCII : StringToASCII  OutputVectorSize=1
  ROT : Outport
  wires:
  Scan String/3 -> DecodeMessage/3(rateOfTurn)
  Compare To Constant/1 -> DecodeMessage/Enable
  Scan String/2 -> String Concatenate/2
  String Concatenate/1 -> DecodeMessage/2(strID)
  ASCII to String3/1 -> Scan String/1
  Timestamp_NMEA/1 -> Select NMEA and Fill Empty Fields/1, SelectTimestamp/1
  DecodeMessage/1(ROT) -> ROT/1
  Byte Unpack2/1 -> DecodeMessage/1(timestamp)  "timestamp"
  SelectTimestamp/1 -> Byte Unpack2/1
  String to ASCII/1 -> Compare To Constant/1
  Select NMEA and Fill Empty Fields/1 -> ASCII to String3/1
  Scan String/1 -> String Concatenate/1
  Scan String/5 -> String to ASCII/1
  Scan String/4 -> DecodeMessage/4(status)

== system NMEA/Decoder/NMEA 0183 Decode VBW ==
  Timestamp_NMEA : Inport
  ASCII to String3 : ASCIIToString
  Byte Unpack2 : etargetslib/Byte Unpack  dimensions={1}  datatypes={'double'}  byteAlign=1
  Compare To Constant : simulink/Logic and Bit Operations/Compare To Constant  relop===  const=uint8(42)  OutDataTypeStr=boolean
  DecodeMessage : Subsystem  TreatAsAtomicUnit=on
  Scan String : ScanString  Format="\"$%c%cVBW,%lf,%lf,%c,%lf,%lf,%c,%lf,%c,%lf,%c%c\""
  Select NMEA and Fill Empty Fields : $bdroot/Details/Select NMEA and Fill Empty Fields
  SelectTimestamp : Selector  IndexOptions=Index vector (dialog)  Indices=1:8  OutputSizes=1
  String Concatenate : StringConcatenate
  String to ASCII : StringToASCII  OutputVectorSize=1
  VBW : Outport
  wires:
  Compare To Constant/1 -> DecodeMessage/Enable
  Scan String/2 -> String Concatenate/2
  String Concatenate/1 -> DecodeMessage/2(strID)
  ASCII to String3/1 -> Scan String/1
  Timestamp_NMEA/1 -> Select NMEA and Fill Empty Fields/1, SelectTimestamp/1
  DecodeMessage/1(VBW) -> VBW/1
  Byte Unpack2/1 -> DecodeMessage/1(timestamp)  "timestamp"
  SelectTimestamp/1 -> Byte Unpack2/1
  String to ASCII/1 -> Compare To Constant/1
  Select NMEA and Fill Empty Fields/1 -> ASCII to String3/1
  Scan String/1 -> String Concatenate/1
  Scan String/3 -> DecodeMessage/3(waterSpeedX)
  Scan String/4 -> DecodeMessage/4(waterSpeedY)
  Scan String/8 -> DecodeMessage/8(strGroundSpeedStatus)
  Scan String/7 -> DecodeMessage/7(groundSpeedY)
  Scan String/6 -> DecodeMessage/6(groundSpeedX)
  Scan String/5 -> DecodeMessage/5(strWaterSpeedStatus)
  Scan String/9 -> DecodeMessage/9(sternTraverseWaterSpeed)
  Scan String/10 -> DecodeMessage/10(sternTraverseWaterSpeedStatus)
  Scan String/11 -> DecodeMessage/11(sternTraverseGroundSpeed)
  Scan String/12 -> DecodeMessage/12(sternTraverseGroundSpeedStatus)
  Scan String/13 -> String to ASCII/1

== system NMEA/Decoder/NMEA 0183 Decode VTG ==
  Timestamp_NMEA : Inport
  ASCII to String3 : ASCIIToString
  Byte Unpack2 : etargetslib/Byte Unpack  dimensions={1}  datatypes={'double'}  byteAlign=1
  Compare To Constant : simulink/Logic and Bit Operations/Compare To Constant  relop===  const=uint8(42)  OutDataTypeStr=boolean
  DecodeMessage : Subsystem  TreatAsAtomicUnit=on
  Scan String : ScanString  Format="\"$%c%cVTG,%lf,T,%lf,M,%lf,N,%lf,K,%c%c\""
  Select NMEA and Fill Empty Fields : $bdroot/Details/Select NMEA and Fill Empty Fields
  SelectTimestamp : Selector  IndexOptions=Index vector (dialog)  Indices=1:8  OutputSizes=1
  String Concatenate : StringConcatenate
  String to ASCII : StringToASCII  OutputVectorSize=1
  VTG : Outport
  wires:
  Scan String/1 -> String Concatenate/1
  Select NMEA and Fill Empty Fields/1 -> ASCII to String3/1
  String to ASCII/1 -> Compare To Constant/1
  SelectTimestamp/1 -> Byte Unpack2/1
  Byte Unpack2/1 -> DecodeMessage/1(timestamp)  "timestamp"
  DecodeMessage/1(VTG) -> VTG/1
  Timestamp_NMEA/1 -> Select NMEA and Fill Empty Fields/1, SelectTimestamp/1
  ASCII to String3/1 -> Scan String/1
  String Concatenate/1 -> DecodeMessage/2(strID)
  Scan String/2 -> String Concatenate/2
  Compare To Constant/1 -> DecodeMessage/Enable
  Scan String/3 -> DecodeMessage/3(trackMadeGoodTrue)
  Scan String/4 -> DecodeMessage/4(trackMadeGoodMagnetic)
  Scan String/5 -> DecodeMessage/5(speedOverGround1)
  Scan String/6 -> DecodeMessage/6(speedOverGround2)
  Scan String/8 -> String to ASCII/1
  Scan String/7 -> DecodeMessage/7(mode)
